simulink model "sim660"  (R2025a)
settings: Solver=ode23s  StartTime=0.0  StopTime=10000  RelTol=1e-3
model workspace (MAT data in the model file):
  op_snapshot1 : opcond.OperatingPoint (value not decoded)
undefined symbols (not defined in the file or in its folder): State132MW, State198MW, State198MW_DELAY
libraries: slpidlib x4, simulink x2, adrc_toolbox_library x1
(part 4 of 5)

== matlab function sim660/Subsystem/MATLAB Function ==
  data: Qc input; Dfw input; dpm output; Dst input; hst input; Drc input; hfw input; pm input; hm input; dhm output; dH output; Vm input; Cm input; eff input; state output; S input; H input; drhodp output; drhodh output; dTdp output; dTdh output; dhVdp output; dhLdp output; drhoVdp output; drhoLdp output; dxdp output; dxdh output
function [dpm,dhm,dH,state,drhodp,drhodh,dTdp,dTdh,dhVdp,dhLdp,drhoVdp,drhoLdp,dxdp,dxdh] = fcn(Qc,Dfw,Dst,hst,Drc,hfw,pm,hm,Vm,Cm,eff,S,H)
%Vm=10;
%Cm=2000;
%eff=0.9;
x=x_ph(pm,hm);
rho=rho_ph(pm,hm);

%%%%%干湿态分别算
if not (x<1 && x>0)
    state=1;
    drhodp=diffx(@rho_ph,pm,hm);
    drhodh=diffy(@rho_ph,pm,hm);
    dTdp=diffx(@T_ph,pm,hm);
    dTdh=diffy(@T_ph,pm,hm);
    A=Vm*drhodp;
    B=Vm*drhodh;
    C=Vm*hm*drhodp+Cm*dTdp;
    D=Vm*hm*drhodh+Vm*rho+Cm*dTdh;
    E=Dfw-Dst;
    F=Dfw*hfw-Dst*hst+Qc;
    out=[A B;C D]\[E;F];
    dpm=out(1);
    dhm=out(2);
    dhVdp=nan;
    dhLdp=nan;
    drhoVdp=nan;
    drhoLdp=nan;
    dxdp=nan;
    dxdh=nan;
    if H>0
        vL=vL_p(pm);
        rhoL=1/vL;
        dH=(-Dst+Dfw+Drc)/(S*rhoL);
    else
    dH=0;
    end
else
    state=x;
    vV=vV_p(pm);
    vL=vL_p(pm);
    rhoV=1/vV;
    rhoL=1/vL;
    hV=hV_p(pm);
    hL=hL_p(pm);
    dTdp=diff1(@Tsat_p,pm);
    dhVdp=dhVdp_p(pm);
    dhLdp=dhLdp_p(pm);
    drhoVdp=diff1(@rho_Vp,pm);
    drhoLdp=diff1(@rho_Lp,pm);
    dxdp=diffx(@x_ph,pm,hm);
    dxdh=diffy(@x_ph,pm,hm);
    %https://www.sciencedirect.com/science/article/pii/S1359431116327727
    Dx=(1-x)*(Dfw+Drc)*eff;
    %A=Vm*(x*drhoVdp+rhoV*dxdp+((1-x)*drhoLdp-rhoL*dxdp)*(1-eff));
    A=Vm*(x*drhoVdp+rhoV*dxdp+((1-x)*drhoLdp-rhoL*dxdp));
    B=Vm*(rhoV*dxdh-rhoL*dxdh);

    %C=Vm*hV*(x*drhoVdp+rhoV*dxdp)+(Vm*hL*((1-x)*drhoLdp-rhoL*dxdp)+Vm*rhoV*x*dhVdp+Vm*rhoL*(1-x)*dhLdp)*(1-eff)+Cm*dTdp;
    C=Vm*hV*(x*drhoVdp+rhoV*dxdp)+(Vm*hL*((1-x)*drhoLdp-rhoL*dxdp)+Vm*rhoV*x*dhVdp+Vm*rhoL*(1-x)*dhLdp)+Cm*dTdp;
    D=Vm*hV*rhoV*dxdh-Vm*hL*rhoL*dxdh;
   
    E=Dfw-Dst+Drc-Dx;
    F=Dfw*hfw+Drc*hL-Dx*hL-Dst*hst+Qc;

    out =[A B;C D]\[E;F];
    dpm=out(1);
    dhm=out(2);
    %dH=(Vm*((1-x)*drhoLdp*dpm-rhoL*dxdh*dhm-rhoL*dxdp*dpm)*eff-Drc)/S;
    dH=(Dx-Drc)/(S*rhoL);
    drhodp=nan;
    drhodh=nan;
    dTdh=nan;

end

%[a b;c d][dpm;dhm]=[e;f]
%out=[dpm;dhm]


end

%%IF97


function rho=rho_Vp(p)
rho=1/vV_p(p);
end
function rho=rho_Lp(p)
rho=1/vL_p(p);
end
function rho=rho_ph(p,h)

rho=1/v_ph(p,h);
end
%% quality
function x = x_ph(p,h)
x = (h - hL_p(p))./(hV_p(p) - hL_p(p));
end

%% stand alone functions
function dhLdp = dhLdp_p(p)
% dhLdp = dhLdp_ph(p)
%   Derivative of enthalpy wrt pressure of saturated liquid, dhLdp [(kJ/kg)/MPa], as a function of pressure, p [MPa]
% based on IAPWS-IF97
% Reference: http://www.iapws.org/
% June 16, 2009
% Mark Mikofski
%% size of inputs
dim = size(p);
dhLdp = NaN(dim);
%% constants and calculated
conversion_factor = 1e-3; % [MPa/(kJ/m^3)]
Tmin = 273.16; % [K] minimum temperature is triple point
TB13 = 623.15; % [K] temperature at boundary between region 1 and 3
pmin = psat_T(Tmin); % [MPa] minimum pressure is 611.657 Pa
pB13sat = psat_T(TB13); % [MPa] saturation pressure at boundary between region 1 and 3, 16.5291643 MPa
pc = 22.064; % [MPa] critical pressure
Tsat = Tsat_p(p); % [K] saturation temperatures
%% valid ranges
valid4a = p>=pmin & p<=pB13sat; % valid range for saturated liquid in region 4a
valid4b = p>pB13sat & p<=pc; % valid range for saturated liquid in region 4b
if any(any(valid4a))
    p4a = p(valid4a);Tsat4a = Tsat(valid4a);
    dhLdp(valid4a) = v1_pT(p4a,Tsat4a).*(1-Tsat4a.*alphav1_pT(p4a,Tsat4a))/conversion_factor + cp1_pT(p4a,Tsat4a).*dTsatdpsat_p(p4a); % [(kJ/kg)/MPa]
end
if any(any(valid4b))
    p4b = p(valid4b); Tsat4b = Tsat(valid4b);v3L = vL_p(p4b);rho3L = 1./v3L;dTsatdpsat4b = dTsatdpsat_p(p4b);
    betap3L = betap3_rhoT(rho3L,Tsat4b);alphap3L = alphap3_rhoT(rho3L,Tsat4b);cv3L = cv3_rhoT(rho3L,Tsat4b);
    dhLdp(valid4b) = (v3L - Tsat4b.*alphap3L./betap3L.*(1 - p4b.*alphap3L.*dTsatdpsat4b))/conversion_factor + (cv3L + p4b.*v3L.*alphap3L).*dTsatdpsat4b;
end
end
function dhVdp = dhVdp_p(p)
% dhVdp = dhVdp_ph(p)
%   Derivative of enthalpy wrt pressure of saturated vapor, dhVdp [(kJ/kg)/MPa], as a function of pressure, p [MPa]
% based on IAPWS-IF97
% Reference: http://www.iapws.org/
% June 16, 2009
% Mark Mikofski
%% size of inputs
dim = size(p);
dhVdp = NaN(dim);
%% constants and calculated
conversion_factor = 1e-3; % [MPa/(kJ/m^3)]
Tmin = 273.16; % [K] minimum temperature is triple point
TB13 = 623.15; % [K] temperature at boundary between region 1 and 3
pmin = psat_T(Tmin); % [MPa] minimum pressure is 611.657 Pa
pB13sat = psat_T(TB13); % [MPa] saturation pressure at boundary between region 1 and 3, 16.5291643 MPa
pc = 22.064; % [MPa] critical pressure
Tsat = Tsat_p(p); % [K] saturation temperatures
%% valid ranges
valid4a = p>=pmin & p<=pB13sat; % valid range for saturated liquid in region 4a
valid4b = p>pB13sat & p<=pc; % valid range for saturated liquid in region 4b
if any(any(valid4a))
    p4a = p(valid4a);Tsat4a = Tsat(valid4a);
    dhVdp(valid4a) = v2_pT(p4a,Tsat4a).*(1-Tsat4a.*alphav2_pT(p4a,Tsat4a))/conversion_factor + cp2_pT(p4a,Tsat4a).*dTsatdpsat_p(p4a); % [(kJ/kg)/MPa]
end
if any(any(valid4b))
    p4b = p(valid4b); Tsat4b = Tsat(valid4b);v3V = vV_p(p4b);rho3V = 1./v3V;dTsatdpsat4b = dTsatdpsat_p(p4b);
    betap3V = betap3_rhoT(rho3V,Tsat4b);alphap3V = alphap3_rhoT(rho3V,Tsat4b);cv3V = cv3_rhoT(rho3V,Tsat4b);
    dhVdp(valid4b) = (v3V - Tsat4b.*alphap3V./betap3V.*(1 - p4b.*alphap3V.*dTsatdpsat4b))/conversion_factor + (cv3V + p4b.*v3V.*alphap3V).*dTsatdpsat4b;
end
end
function v = vL_p(p)
% v = vL_p(p)
%   Specific volume of saturated liquid, v [m^3/kg], as a function of pressure, p [MPa]
% based on IAPWS-IF97
% Reference: http://www.iapws.org/
% June 5, 2009
% Mark Mikofski
%% size of inputs
dim = size(p);
v = NaN(dim);
%% constants and calculated
Tmin = 273.16; % [K] minimum temperature is triple point
TB13 = 623.15; % [K] temperature at boundary between region 1 and 3
pmin = psat_T(Tmin); % [MPa] minimum pressure is 611.657 Pa
pB13sat = psat_T(TB13); % [MPa] saturation pressure at boundary between region 1 and 3, 16.5291643 MPa
pc = 22.064; % [MPa] critical pressure
Tsat = Tsat_p(p); % [K] saturation temperatures
%% valid ranges
valid4a = p>=pmin & p<=pB13sat; % valid range for saturated liquid in region 4a
valid4b = p>pB13sat & p<=pc; % valid range for saturated liquid in region 4b
if any(any(valid4a))
    v(valid4a) = v1_pT(p(valid4a),Tsat(valid4a)); % [kJ/kg] saturated liquid enthalpies in region 1
end
if any(any(valid4b))
    p3cd = 19.00881189173929; % [MPa] pressure given by T3cd_p(p) = Tsat_p(p)
    valid3c = p>pB13sat & p<=p3cd;
    p3q = psat_T(643.15); % [MPa] 21.0434 MPa
    valid3s = p>p3cd & p<=p3q;
    p3y = 21.93161551; % [MPa] p3sat_v(0.00264 m^3/kg), n.b. p3sat_v is not an available function yet
    valid3u = p>p3q & p<=p3y;
    valid3y = p>p3y & p<=pc;
    if any(any(valid3c))
        v(valid3c) = v3c_pT(p(valid3c),Tsat(valid3c));
    end
    if any(any(valid3s))
        v(valid3s) = v3s_pT(p(valid3s),Tsat(valid3s));
    end
    if any(any(valid3u))
        v(valid3u) = v3u_pT(p(valid3u),Tsat(valid3u));
    end
    if any(any(valid3y))
        v(valid3y) = v3y_pT(p(valid3y),Tsat(valid3y));
    end
end
end
function v = vV_p(p)
% v = vV_p(p)
%   Specific volume of saturated vapor, v [m^3/kg], as a function of pressure, p [MPa]
% based on IAPWS-IF97
% Reference: http://www.iapws.org/
% June 5, 2009
% Mark Mikofski
%% size of inputs
dim = size(p);
v = NaN(dim);
%% constants and calculated
Tmin = 273.16; % [K] minimum temperature is triple point
TB13 = 623.15; % [K] temperature at boundary between region 1 and 3
pmin = psat_T(Tmin); % [MPa] minimum pressure is 611.657 Pa
pB13sat = psat_T(TB13); % [MPa] saturation pressure at boundary between region 1 and 3, 16.5291643 MPa
pc = 22.064; % [MPa] critical pressure
Tsat = Tsat_p(p); % [K] saturation temperatures
%% valid ranges
valid4a = p>=pmin & p<=pB13sat; % valid range for saturated liquid in region 4a
valid4b = p>pB13sat & p<=pc; % valid range for saturated liquid in region 4b
if any(any(valid4a))
    v(valid4a) = v2_pT(p(valid4a),Tsat(valid4a)); % [kJ/kg] saturated liquid enthalpies in region 2
end
if any(any(valid4b))
    valid3t = p>pB13sat & p<=20.5;
    p3q = psat_T(643.15); % [MPa] 21.0434 MPa
    valid3r = p>20.5 & p<=p3q;
    p3z = 21.90096265; % [MPa] p3sat_v(0.00385 m^3/kg), n.b. p3sat_v is not an available function yet
    valid3x = p>p3q & p<=p3z;
    valid3z = p>p3z & p<=pc;
    if any(any(valid3t))
        v(valid3t) = v3t_pT(p(valid3t),Tsat(valid3t));
    end
    if any(any(valid3r))
        v(valid3r) = v3r_pT(p(valid3r),Tsat(valid3r));
    end
    if any(any(valid3x))
        v(valid3x) = v3x_pT(p(valid3x),Tsat(valid3x));
    end
    if any(any(valid3z))
        v(valid3z) = v3z_pT(p(valid3z),Tsat(valid3z));
    end
end
end
function h = hL_p(p)
% h = hL_p(p)
%   Enthalpy of saturated liquid, h [kJ/kg], as a function of pressure, p [MPa]
% based on IAPWS-IF97
% Reference: http://www.iapws.org/
% June 2, 2009
% Mark Mikofski
%% size of inputs
dim = size(p);
h = NaN(dim);
%% constants and calculated
Tmin = 273.16; % [K] minimum temperature is triple point
TB13 = 623.15; % [K] temperature at boundary between region 1 and 3
pmin = psat_T(Tmin); % [MPa] minimum pressure is 611.657 Pa
pB13sat = psat_T(TB13); % [MPa] saturation pressure at boundary between region 1 and 3, 16.5291643 MPa
pc = 22.064; % [MPa] critical pressure
Tsat = Tsat_p(p); % [K] saturation temperatures
%% valid ranges
valid4a = p>=pmin & p<=pB13sat; % valid range for saturated liquid in region 4a
valid4b = p>pB13sat & p<=pc; % valid range for saturated liquid in region 4b
if any(any(valid4a))
    h(valid4a) = h1_pT(p(valid4a),Tsat(valid4a)); % [kJ/kg] saturated liquid enthalpies in region 1
end
if any(any(valid4b))
    h(valid4b) = h3_rhoT(1./vL_p(p(valid4b)),Tsat(valid4b));
end
end
function h = hV_p(p)
% h = hV_p(p)
%   Enthalpy of saturated vapor, h [kJ/kg], as a function of pressure, p [MPa]
% based on IAPWS-IF97
% Reference: http://www.iapws.org/
% June 2, 2009
% Mark Mikofski
%% size of inputs
dim = size(p);
h = NaN(dim);
%% constants and calculated
Tmin = 273.16; % [K] minimum temperature is triple point
TB13 = 623.15; % [K] temperature at boundary between region 1 and 3
pmin = psat_T(Tmin); % [MPa] minimum pressure is 611.657 Pa
pB13sat = psat_T(TB13); % [MPa] saturation pressure at boundary between region 1 and 3, 16.5291643 MPa
pc = 22.064; % [MPa] critical pressure
Tsat = Tsat_p(p); % [K] saturation temperatures
%% valid ranges
valid4a = p>=pmin & p<=pB13sat; % valid range for saturated liquid in region 4a
valid4b = p>pB13sat & p<=pc; % valid range for saturated liquid in region 4b
if any(any(valid4a))
    h(valid4a) = h2_pT(p(valid4a),Tsat(valid4a)); % [kJ/kg] saturated liquid enthalpies in region 2
end
if any(any(valid4b))
    h(valid4b) = h3_rhoT(1./vV_p(p(valid4b)),Tsat(valid4b));
end
end
function T = T_ph(p,h)
% T = T_ph(p,h)
%   Temperature of liquid, vapor or mixture, T [K], as functions of pressure, p [MPa], and enthalpy, h [kJ/kg]
% based on IAPWS-IF97
% Reference: http://www.iapws.org/
% June 2, 2009
% Mark Mikofski
%% size of inputs
dim = size(p);
initnan = NaN(dim);
T = initnan;
%% constants and calculated scalars
Tmin = 273.16; % [K] minimum temperature is triple point
T2bcsat = 554.485; % [K] saturation temperature at 5.85 kJ/kg/K isentropic line between region 2b and 2c
TB13 = 623.15; % [K] temperature at boundary between region 1 and 3
Tmax = 1073.15; % [K] maximum temperature
pmin = psat_T(Tmin); % [MPa] minimum pressure is 611.657 Pa
p2ab = 4; % [MPa] pressure along boundary between region 2a and 2b
p2bcsat = psat_T(T2bcsat); % [MPa] saturation pressure at 5.85 kJ/kg/K isentropic line between region 2b and 2c
pB13sat = psat_T(TB13); % [MPa] saturation pressure at boundary between region 1 and 3, 16.5291643 MPa
pmax = 100; % [MPa] maximum pressure
h1B13L = h1_pT(pB13sat,TB13); % [kJ/kg] saturated liquid enthalpy at boundary between region 1, region 3 and region 4
h2B13V = h2_pT(pB13sat,TB13); % [kJ/kg] saturated vapor enthalpy at boundary between region 2, region 3 and region 4
%% calculated matrices
Tsat = Tsat_p(p); % [K] saturation temperatures
h1min = initnan;h2max = initnan;valid = p>=pmin & p<=pmax;pvalid = p(valid); % initialize matricies with NaN and set valid range of parameters
if any(any(valid))
    Tmin = Tmin*ones(dim);Tmax = Tmax*ones(dim); % copy to matrix of size dim
    h1min(valid) = h1_pT(pvalid,Tmin(valid)); % [kJ/kg] minimum enthalpies
    h2max(valid) = h2_pT(pvalid,Tmax(valid)); % [kJ/kg] maximum enthalpies in region 2
end
h1L = initnan;h2V = initnan;valid = p>=pmin & p<=pB13sat;pvalid = p(valid); % initialize matricies with NaN and set valid range of parameters
if any(any(valid))
    h1L(valid) = h1_pT(pvalid,Tsat(valid)); % [kJ/kg] saturated liquid enthalpies in region 1
    h2V(valid) = h2_pT(pvalid,Tsat(valid)); % [kJ/kg] saturated vapor enthalpies in region 2
end
h1B13 = initnan;h3ab = initnan;h2B23 = initnan;valid = p>=pB13sat & p<=pmax;pvalid = p(valid); % initialize matricies with NaN and set valid range of parameters
if any(any(valid))
    TB13 = TB13*ones(dim); % copy to matrix of size dim
    h1B13(valid) = h1_pT(pvalid,TB13(valid)); % [kJ/kg] enthalpies on boundary between region 1 and region 3
    h3ab(valid) = h3ab_p(pvalid); % [kJ/kg] enthalpies on critical entropy isentropic line between regions 3a and region 3b
    h2B23(valid) = h2_pT(pvalid,TB23_p(pvalid)); % [kJ/kg] enthalpies on boundary between region 2 and region 3
end
h2bc = initnan;valid = p>=p2bcsat & p<=pmax; % initialize matricies with NaN and set valid range of parameters
h2bc(valid) = h2bc_p(p(valid)); % [kJ/kg] enthalpies on boundary between region 2b and 2c
p3sat = pB13sat*ones(dim);valid = h>=h1B13L & h<=h2B13V; % % do NOT use NaN to initialize p3sat, b/c for h<h1B13L or h>h2B13V p>NaN = 0, instead use pB13sat
if any(any(valid))
    p3sat(valid) = p3sat_h(h(valid)); % [MPa] saturation pressure on boundary between region 3 and 4
end
%% valid ranges
valid1 = (p>=pmin & p<=pB13sat & h>=h1min & h<=h1L) | (p>pB13sat & p<=pmax & h>=h1min & h<=h1B13); % valid range for region 1
valid2a = p>=pmin & p<=p2ab & h>h2V & h<=h2max; % valid range for region 2a
valid2b = (p>p2ab & p<=p2bcsat & h>h2V & h<=h2max) | (p>p2bcsat & p<=pmax & h>h2bc & h<=h2max); % valid range for region 2b
valid2c = (p>p2bcsat & p<=pB13sat & h>h2V & h<=h2bc) | (p>pB13sat & p<=pmax & h>h2B23 & h<=h2bc); % valid range for region 2c
valid3a = p>p3sat & p<=pmax & h>h1B13 & h<=h3ab; % valid range for region 3a
valid3b = p>p3sat & p<=pmax & h>h3ab & h<=h2B23; % valid range for region 3b
valid4 = (p>=pmin & p<=pB13sat & h>h1L & h<=h2V) | (p>pB13sat & p<=p3sat & h>h1B13L & h<=h2B13V); % valid range for region 4
if any(any(valid1))
    T(valid1) = T1_ph(p(valid1),h(valid1));
end
if any(any(valid2a))
    T(valid2a) = T2a_ph(p(valid2a),h(valid2a));
end
if any(any(valid2b))
    T(valid2b) = T2b_ph(p(valid2b),h(valid2b));
end
if any(any(valid2c))
    T(valid2c) = T2c_ph(p(valid2c),h(valid2c));
end
if any(any(valid3a))
    T(valid3a) = T3a_ph(p(valid3a),h(valid3a));
end
if any(any(valid3b))
    T(valid3b) = T3b_ph(p(valid3b),h(valid3b));
end
if any(any(valid4))
    T(valid4) = Tsat(valid4);
end
end
function v = v_ph(p,h)
% v = v_ph(p,h)
%   Specific volume of liquid, vapor or mixture, v [m^3/kg], as functions of pressure, p [MPa], and enthalpy, h [kJ/kg]
% based on IAPWS-IF97
% Reference: http://www.iapws.org/
% June 1, 2009
% Mark Mikofski
%% size of inputs
dim = size(p);
initnan = NaN(dim);
v = initnan;
%% constants and calculated scalars
Tmin = 273.16; % [K] minimum temperature is triple point
T2bcsat = 554.485; % [K] saturation temperature at 5.85 kJ/kg/K isentropic line between region 2b and 2c
TB13 = 623.15; % [K] temperature at boundary between region 1 and 3
Tmax = 1073.15; % [K] maximum temperature
pmin = psat_T(Tmin); % [MPa] minimum pressure is 611.657 Pa
p2ab = 4; % [MPa] pressure along boundary between region 2a and 2b
p2bcsat = psat_T(T2bcsat); % [MPa] saturation pressure at 5.85 kJ/kg/K isentropic line between region 2b and 2c
pB13sat = psat_T(TB13); % [MPa] saturation pressure at boundary between region 1 and 3, 16.5291643 MPa
pmax = 100; % [MPa] maximum pressure
h1B13L = h1_pT(pB13sat,TB13); % [kJ/kg] saturated liquid enthalpy at boundary between region 1, region 3 and region 4
h2B13V = h2_pT(pB13sat,TB13); % [kJ/kg] saturated vapor enthalpy at boundary between region 2, region 3 and region 4
%% calculated matrices
Tsat = Tsat_p(p); % [K] saturation temperatures
h1min = initnan;h2max = initnan;valid = p>=pmin & p<=pmax;pvalid = p(valid); % initialize matricies with NaN and set valid range of parameters
if any(any(valid))
    Tmin = Tmin*ones(dim);Tmax = Tmax*ones(dim); % copy to matrix of size dim
    h1min(valid) = h1_pT(pvalid,Tmin(valid)); % [kJ/kg] minimum enthalpies
    h2max(valid) = h2_pT(pvalid,Tmax(valid)); % [kJ/kg] maximum enthalpies in region 2
end
h1L = initnan;h2V = initnan;valid = p>=pmin & p<=pB13sat;pvalid = p(valid); % initialize matricies with NaN and set valid range of parameters
if any(any(valid))
    h1L(valid) = h1_pT(pvalid,Tsat(valid)); % [kJ/kg] saturated liquid enthalpies in region 1
    h2V(valid) = h2_pT(pvalid,Tsat(valid)); % [kJ/kg] saturated vapor enthalpies in region 2
end
h1B13 = initnan;h3ab = initnan;h2B23 = initnan;valid = p>=pB13sat & p<=pmax;pvalid = p(valid); % initialize matricies with NaN and set valid range of parameters
if any(any(valid))
    TB13 = TB13*ones(dim); % copy to matrix of size dim
    h1B13(valid) = h1_pT(pvalid,TB13(valid)); % [kJ/kg] enthalpies on boundary between region 1 and region 3
    h3ab(valid) = h3ab_p(pvalid); % [kJ/kg] enthalpies on critical entropy isentropic line between regions 3a and region 3b
    h2B23(valid) = h2_pT(pvalid,TB23_p(pvalid)); % [kJ/kg] enthalpies on boundary between region 2 and region 3
end
h2bc = initnan;valid = p>=p2bcsat & p<=pmax; % initialize matricies with NaN and set valid range of parameters
h2bc(valid) = h2bc_p(p(valid)); % [kJ/kg] enthalpies on boundary between region 2b and 2c
p3sat = pB13sat*ones(dim);valid = h>=h1B13L & h<=h2B13V; % % do NOT use NaN to initialize p3sat, b/c for h<h1B13L or h>h2B13V p>NaN = 0, instead use pB13sat
if any(any(valid))
    p3sat(valid) = p3sat_h(h(valid)); % [MPa] saturation pressure on boundary between region 3 and 4
end
%% valid ranges
valid1 = (p>=pmin & p<=pB13sat & h>=h1min & h<=h1L) | (p>pB13sat & p<=pmax & h>=h1min & h<=h1B13); % valid range for region 1
valid2a = p>=pmin & p<=p2ab & h>h2V & h<=h2max; % valid range for region 2a
valid2b = (p>p2ab & p<=p2bcsat & h>h2V & h<=h2max) | (p>p2bcsat & p<=pmax & h>h2bc & h<=h2max); % valid range for region 2b
valid2c = (p>p2bcsat & p<=pB13sat & h>h2V & h<=h2bc) | (p>pB13sat & p<=pmax & h>h2B23 & h<=h2bc); % valid range for region 2c
valid3a = p>p3sat & p<=pmax & h>h1B13 & h<=h3ab; % valid range for region 3a
valid3b = p>p3sat & p<=pmax & h>h3ab & h<=h2B23; % valid range for region 3b
valid4a = p>=pmin & p<=pB13sat & h>h1L & h<=h2V; % valid range for region 4a
valid4b = p>pB13sat & p<=p3sat & h>h1B13L & h<=h2B13V; % valid range for region 4b
if any(any(valid1))
    p1 = p(valid1);
    v(valid1) = v1_pT(p1,T1_ph(p1,h(valid1)));
end
if any(any(valid2a))
    p2a = p(valid2a);
    v(valid2a) = v2_pT(p2a,T2a_ph(p2a,h(valid2a)));
end
if any(any(valid2b))
    p2b = p(valid2b);
    v(valid2b) = v2_pT(p2b,T2b_ph(p2b,h(valid2b)));
end
if any(any(valid2c))
    p2c = p(valid2c);
    v(valid2c) = v2_pT(p2c,T2c_ph(p2c,h(valid2c)));
end
if any(any(valid3a))
    v(valid3a) = v3a_ph(p(valid3a),h(valid3a));
end
if any(any(valid3b))
    v(valid3b) = v3b_ph(p(valid3b),h(valid3b));
end
if any(any(valid4a))
    p4a = p(valid4a);Tsat4a = Tsat(valid4a);h1L4a = h1L(valid4a);
    x = (h(valid4a)-h1L4a)./(h2V(valid4a)-h1L4a); % quality
    v1L = v1_pT(p4a,Tsat4a); % [m^3/kg] saturated liquid specific volumes
    v2V = v2_pT(p4a,Tsat4a); % [m^3/kg] saturated vapor specific volumes
    v(valid4a) = v1L + x.*(v2V - v1L);
end
if any(any(valid4b))
    p4b = p(valid4b); Tsat4b = Tsat(valid4b);
    v3L = vL_p(p4b); v3V = vV_p(p4b);
    h3L = h3_rhoT(1./v3L,Tsat4b);
    h3V = h3_rhoT(1./v3V,Tsat4b);
    x = (h(valid4b)-h3L)./(h3V-h3L); % quality
    v(valid4b) = v3L + x.*(v3V - v3L);
end
end
function p = psat_T(T)
% p = psat_T(T)
%   Pressure of saturated liquid, mixture or steam, p [MPa], as a function of temperature, T [K]
% based on IAPWS-IF97
% Reference: http://www.iapws.org/
% June 9, 2009
% Mark Mikofski
dim = size(T);
p = NaN(dim);
Tmin = 273.16; % [K] minimum temperature is triple point
Tc = 647.096; % [K] critical point temperature
valid = T>=Tmin & T<=Tc;
pstar = 1; % [Mpa]
Tstar = 1; % [K]
n = [1167.05214527670;-724213.167032060;-17.0738469400920;12020.8247024700;-3232555.03223330;14.9151086135300; ...
    -4823.26573615910;405113.405420570;-0.238555575678490;650.175348447980];
upsilon = T(valid)/Tstar + n(9)./(T(valid)/Tstar-n(10));
A = (upsilon + n(1)).*upsilon + n(2); % use Horner's Method to speed up calculations
B = (n(3)*upsilon + n(4)).*upsilon + n(5); % use Horner's Method to speed up calculations
C = (n(6)*upsilon + n(7)).*upsilon + n(8); % use Horner's Method to speed up calculations
beta = 2*C./(-B + (B.^2 - 4*A.*C).^0.5);
p(valid) = (beta.^4) * pstar;
end
function T = Tsat_p(p)
% T = Tsat_p(p)
%   Temperature of saturated liquid, mixture or steam, T [K], as a function of temperature, p [MPa]
% based on IAPWS-IF97
% Reference: http://www.iapws.org/
% June 9, 2009
% Mark Mikofski
dim = size(p);
T = NaN(dim);
Tmin = 273.16; % [K] minimum temperature is triple point
pmin = psat_T(Tmin); % [MPa] minimum pressure is 611.657 Pa
pc = 22.064; % [MPa] critical pressure
valid = p>=pmin & p<=pc; % initialize matricies with NaN and set valid range of parameters
pstar = 1; % [Mpa]
Tstar = 1; % [K]
n = [1167.05214527670;-724213.167032060;-17.0738469400920;12020.8247024700;-3232555.03223330;14.9151086135300; ...
    -4823.26573615910;405113.405420570;-0.238555575678490;650.175348447980];
beta = (p(valid)/pstar).^0.25;
E = (beta + n(3)).*beta + n(6); % use Horner's Method to speed up calculations
F = (n(1)*beta + n(4)).*beta + n(7); % use Horner's Method to speed up calculations
G = (n(2)*beta + n(5)).*beta + n(8); % use Horner's Method to speed up calculations
D = 2*G./(-F - (F.^2 - 4*E.*G).^0.5);
n11 = n(10) + D;
theta = (n11 - (n11.^2 - 4*(n(9) + n(10)*D)).^0.5)/2;
T(valid) = theta*Tstar;
end
%% basic and fundamental functions
function h = h1_pT(p,T) % [kJ/kg]
R = 0.461526; % [kJ/kg/K] specific gas constant
Tstar = 1386; % [K]
h = R*Tstar*dgammadtau1_pT(p,T);
end
function h = h2_pT(p,T) % [kJ/kg]
R = 0.461526; % [kJ/kg/K] specific gas constant
Tstar = 540; % [K]
h = R*Tstar*dgammadtau2_pT(p,T);
end
function h = h3_rhoT(rho,T)
R = 0.461526; % [kJ/kg/K] specific gas constant
Tc = 647.096; % [K] critical point temperature
rhoc = 322; % [kg/m^3] critical point density
delta = rho/rhoc;
h = R*(Tc*dphidtau3_rhoT(rho,T) + T.*delta.*dphiddelta3_rhoT(rho,T));
end
function v = v1_pT(p,T) % [m^3/kg]
R = 0.461526; % [kJ/kg/K] specific gas constant
conversion_factor = 1e-3; % [MPa/(kJ/m^3)]
pstar = 16.53; % [MPa]
v = conversion_factor*R*T/pstar.*dgammadpi1_pT(p,T);
end
function v = v2_pT(p,T) % [m^3/kg]
R = 0.461526; % [kJ/kg/K] specific gas constant
conversion_factor = 1e-3; % [MPa/(kJ/m^3)]
pstar = 1; % [MPa]
v = conversion_factor*R*T/pstar.*dgammadpi2_pT(p,T);
end
function cp = cp1_pT(p,T) % [kJ/kg/K]
R = 0.461526; % [kJ/kg/K] specific gas constant
Tstar = 1386; % [K]
tau = Tstar./T;
cp = -R*tau.^2.*dgammadtautau1_pT(p,T);
end
function cp = cp2_pT(p,T) % [kJ/kg/K]
R = 0.461526; % [kJ/kg/K] specific gas constant
Tstar = 540; % [K]
tau = Tstar./T;
cp = -R*tau.^2.*dgammadtautau2_pT(p,T);
end
function cv = cv3_rhoT(rho,T)
R = 0.461526; % [kJ/kg/K] specific gas constant
Tc = 647.096; % [K] critical point temperature
tau = Tc./T;
cv = R*(-tau.^2.*dphidtautau3_rhoT(rho,T));
end
function alphav = alphav1_pT(p,T)
Tstar = 1386; % [K]
tau = Tstar./T;
alphav = (1-tau.*dgammadpitau1_pT(p,T)./dgammadpi1_pT(p,T))./T;
end
function alphav = alphav2_pT(p,T)
Tstar = 540; % [K]
tau = Tstar./T;
alphav = (1-tau.*dgammadpitau2_pT(p,T)./dgammadpi2_pT(p,T))./T;
end
function alphap = alphap3_rhoT(rho,T)
Tc = 647.096; % [K] critical point temperature
tau = Tc./T;
alphap = (1-tau.*dphiddeltatau3_rhoT(rho,T)./dphiddelta3_rhoT(rho,T))./T;
end
function betap = betap3_rhoT(rho,T)
rhoc = 322; % [kg/m^3] critical point density
delta = rho/rhoc;
betap = rho.*(2+delta.*dphiddeltadelta3_rhoT(rho,T)./dphiddelta3_rhoT(rho,T));
end
function dgammadtau = dgammadtau1_pT(p,T)
dim = length(p);
pstar = 16.53; % [MPa]
Tstar = 1386; % [K]
pi = p/pstar;
tau = Tstar./T;
I = [0,0,0,0,0,0,0,0,1,1,1,1,1,1,2,2,2,2,2,3,3,3,4,4,4,5,8,8,21,23,29,30,31,32];
J = [-2,-1,0,1,2,3,4,5,-9,-7,-1,0,1,3,-3,0,1,3,17,-4,0,6,-5,-2,10,-8,-11,-6,-29,-31,-38,-39,-40,-41];
n = [0.146329712131670,-0.845481871691140,-3.75636036720400,3.38551691683850,-0.957919633878720,0.157720385132280, ...
    -0.0166164171995010,0.000812146299835680,0.000283190801238040,-0.000607063015658740,-0.0189900682184190, ...
    -0.0325297487705050,-0.0218417171754140,-5.28383579699300e-05,-0.000471843210732670,-0.000300017807930260, ...
    4.76613939069870e-05,-4.41418453308460e-06,-7.26949962975940e-16,-3.16796448450540e-05,-2.82707979853120e-06, ...
    -8.52051281201030e-10,-2.24252819080000e-06,-6.51712228956010e-07,-1.43417299379240e-13,-4.05169968601170e-07, ...
    -1.27343017416410e-09,-1.74248712306340e-10,-6.87621312955310e-19,1.44783078285210e-20,2.63357816627950e-23, ...
    -1.19476226400710e-23,1.82280945814040e-24,-9.35370872924580e-26];
Nterms = 34;
I = ones(dim,1)*I;
J = ones(dim,1)*J;
n = ones(dim,1)*n;
pi = pi*ones(1,Nterms);
tau = tau*ones(1,Nterms);
dgammadtau = sum(n.*(7.1-pi).^I.*J.*(tau-1.222).^(J-1),2);
end
function dgammadpi = dgammadpi1_pT(p,T)
dim = length(p);
pstar = 16.53; % [MPa]
Tstar = 1386; % [K]
pi = p/pstar;
tau = Tstar./T;
I = [0,0,0,0,0,0,0,0,1,1,1,1,1,1,2,2,2,2,2,3,3,3,4,4,4,5,8,8,21,23,29,30,31,32];
J = [-2,-1,0,1,2,3,4,5,-9,-7,-1,0,1,3,-3,0,1,3,17,-4,0,6,-5,-2,10,-8,-11,-6,-29,-31,-38,-39,-40,-41];
n = [0.146329712131670,-0.845481871691140,-3.75636036720400,3.38551691683850,-0.957919633878720,0.157720385132280, ...
    -0.0166164171995010,0.000812146299835680,0.000283190801238040,-0.000607063015658740,-0.0189900682184190, ...
    -0.0325297487705050,-0.0218417171754140,-5.28383579699300e-05,-0.000471843210732670,-0.000300017807930260, ...
    4.76613939069870e-05,-4.41418453308460e-06,-7.26949962975940e-16,-3.16796448450540e-05,-2.82707979853120e-06, ...
    -8.52051281201030e-10,-2.24252819080000e-06,-6.51712228956010e-07,-1.43417299379240e-13,-4.05169968601170e-07, ...
    -1.27343017416410e-09,-1.74248712306340e-10,-6.87621312955310e-19,1.44783078285210e-20,2.63357816627950e-23, ...
    -1.19476226400710e-23,1.82280945814040e-24,-9.35370872924580e-26];
Nterms = 34;
I = ones(dim,1)*I;
J = ones(dim,1)*J;
n = ones(dim,1)*n;
pi = pi*ones(1,Nterms);
tau = tau*ones(1,Nterms);
dgammadpi = sum(-n.*I.*(7.1-pi).^(I-1).*(tau-1.222).^J,2);
end
function dgammadtautau = dgammadtautau1_pT(p,T)
dim = length(p);
pstar = 16.53; % [MPa]
Tstar = 1386; % [K]
pi = p/pstar;
tau = Tstar./T;
I = [0,0,0,0,0,0,0,0,1,1,1,1,1,1,2,2,2,2,2,3,3,3,4,4,4,5,8,8,21,23,29,30,31,32];
J = [-2,-1,0,1,2,3,4,5,-9,-7,-1,0,1,3,-3,0,1,3,17,-4,0,6,-5,-2,10,-8,-11,-6,-29,-31,-38,-39,-40,-41];
n = [0.146329712131670,-0.845481871691140,-3.75636036720400,3.38551691683850,-0.957919633878720,0.157720385132280, ...
    -0.0166164171995010,0.000812146299835680,0.000283190801238040,-0.000607063015658740,-0.0189900682184190, ...
    -0.0325297487705050,-0.0218417171754140,-5.28383579699300e-05,-0.000471843210732670,-0.000300017807930260, ...
    4.76613939069870e-05,-4.41418453308460e-06,-7.26949962975940e-16,-3.16796448450540e-05,-2.82707979853120e-06, ...
    -8.52051281201030e-10,-2.24252819080000e-06,-6.51712228956010e-07,-1.43417299379240e-13,-4.05169968601170e-07, ...
    -1.27343017416410e-09,-1.74248712306340e-10,-6.87621312955310e-19,1.44783078285210e-20,2.63357816627950e-23, ...
    -1.19476226400710e-23,1.82280945814040e-24,-9.35370872924580e-26];
Nterms = 34;
I = ones(dim,1)*I;
J = ones(dim,1)*J;
n = ones(dim,1)*n;
pi = pi*ones(1,Nterms);
tau = tau*ones(1,Nterms);
dgammadtautau = sum(n.*(7.1-pi).^I.*J.*(J-1).*(tau-1.222).^(J-2),2);
end
function dgammadpitau = dgammadpitau1_pT(p,T)
dim = length(p);
pstar = 16.53; % [MPa]
Tstar = 1386; % [K]
pi = p/pstar;
tau = Tstar./T;
I = [0,0,0,0,0,0,0,0,1,1,1,1,1,1,2,2,2,2,2,3,3,3,4,4,4,5,8,8,21,23,29,30,31,32];
J = [-2,-1,0,1,2,3,4,5,-9,-7,-1,0,1,3,-3,0,1,3,17,-4,0,6,-5,-2,10,-8,-11,-6,-29,-31,-38,-39,-40,-41];
n = [0.146329712131670,-0.845481871691140,-3.75636036720400,3.38551691683850,-0.957919633878720,0.157720385132280, ...
    -0.0166164171995010,0.000812146299835680,0.000283190801238040,-0.000607063015658740,-0.0189900682184190, ...
    -0.0325297487705050,-0.0218417171754140,-5.28383579699300e-05,-0.000471843210732670,-0.000300017807930260, ...
    4.76613939069870e-05,-4.41418453308460e-06,-7.26949962975940e-16,-3.16796448450540e-05,-2.82707979853120e-06, ...
    -8.52051281201030e-10,-2.24252819080000e-06,-6.51712228956010e-07,-1.43417299379240e-13,-4.05169968601170e-07, ...
    -1.27343017416410e-09,-1.74248712306340e-10,-6.87621312955310e-19,1.44783078285210e-20,2.63357816627950e-23, ...
    -1.19476226400710e-23,1.82280945814040e-24,-9.35370872924580e-26];
Nterms = 34;
I = ones(dim,1)*I;
J = ones(dim,1)*J;
n = ones(dim,1)*n;
pi = pi*ones(1,Nterms);
tau = tau*ones(1,Nterms);
dgammadpitau = sum(-n.*I.*(7.1-pi).^(I-1).*J.*(tau-1.222).^(J-1),2);
end
function dgammadtau = dgammadtau2_pT(p,T)
dim = length(p);
pstar = 1; % [MPa] scaling pressure for nondimensional pressure, pi
Tstar = 540; % [K] scaling temperature for nondimensional temperature substitution variable
pi = p/pstar; % nondimensional pressure
tau = Tstar./T; % temperature substitution variable
%% ideal part
J0 = [0,1,-5,-4,-3,-2,-1,2,3]; % ideal part exponenets
n0 = [-9.69276865002170,10.0866559680180,-0.00560879112830200,0.0714527380814550,-0.407104982239280,1.42408191714440, ...
    -4.38395113194500,-0.284086324607720,0.0212684637533070];
N0terms = 9; % number of ideal terms in summation
J0 = ones(dim,1)*J0;
n0 = ones(dim,1)*n0;
tau0 = tau*ones(1,N0terms);
dgammadtau0 = sum(n0.*J0.*tau0.^(J0-1),2); % index sums of valid inputs into corresponding location in output array
%% residual part
IR = [1,1,1,1,1,2,2,2,2,2,3,3,3,3,3,4,4,4,5,6,6,6,7,7,7,8,8,9,10,10,10,16,16,18,20,20,20,21,22,23,24,24,24];
JR = [0,1,2,3,6,1,2,4,7,36,0,1,3,6,35,1,2,3,7,3,16,35,0,11,25,8,36,13,4,10,14,29,50,57,20,35,48,21,53,39,26,40,58];
nR = [-0.00177317424732130,-0.0178348622923580,-0.0459960136963650,-0.0575812590834320,-0.0503252787279300, ...
    -3.30326416702030e-05,-0.000189489875163150,-0.00393927772433550,-0.0437972956505730,-2.66745479140870e-05, ...
    2.04817376923090e-08,4.38706672844350e-07,-3.22776772385700e-05,-0.00150339245421480,-0.0406682535626490, ...
    -7.88473095593670e-10,1.27907178522850e-08,4.82253727185070e-07,2.29220763376610e-06,-1.67147664510610e-11, ...
    -0.00211714723213550,-23.8957419341040,-5.90595643242700e-18,-1.26218088991010e-06,-0.0389468424357390, ...
    1.12562113604590e-11,-8.23113408979980,1.98097128020880e-08,1.04069652101740e-19,-1.02347470959290e-13, ...
    -1.00181793795110e-09,-8.08829086469850e-11,0.106930318794090,-0.336622505741710,8.91858453554210e-25, ...
    3.06293168762320e-13,-4.20024676982080e-06,-5.90560296856390e-26,3.78269476134570e-06,-1.27686089346810e-15, ...
    7.30876105950610e-29,5.54147153507780e-17,-9.43697072412100e-07];
NRterms = 43;
IR = ones(dim,1)*IR;
JR = ones(dim,1)*JR;
nR = ones(dim,1)*nR;
pi = pi*ones(1,NRterms);
tauR = tau*ones(1,NRterms);
dgammadtauR = sum(nR.*pi.^IR.*JR.*(tauR-0.5).^(JR-1),2);
dgammadtau = dgammadtau0 + dgammadtauR;
end
function dgammadpi = dgammadpi2_pT(p,T)
dim = length(p);
pstar = 1; % [MPa] scaling pressure for nondimensional pressure, pi
Tstar = 540; % [K] scaling temperature for nondimensional temperature substitution variable
pi = p/pstar; % nondimensional pressure
tau = Tstar./T; % temperature substitution variable
%% ideal part
dgammadpi0 = 1./pi;
%% residual part
IR = [1,1,1,1,1,2,2,2,2,2,3,3,3,3,3,4,4,4,5,6,6,6,7,7,7,8,8,9,10,10,10,16,16,18,20,20,20,21,22,23,24,24,24];
JR = [0,1,2,3,6,1,2,4,7,36,0,1,3,6,35,1,2,3,7,3,16,35,0,11,25,8,36,13,4,10,14,29,50,57,20,35,48,21,53,39,26,40,58];
nR = [-0.00177317424732130,-0.0178348622923580,-0.0459960136963650,-0.0575812590834320,-0.0503252787279300, ...
    -3.30326416702030e-05,-0.000189489875163150,-0.00393927772433550,-0.0437972956505730,-2.66745479140870e-05, ...
    2.04817376923090e-08,4.38706672844350e-07,-3.22776772385700e-05,-0.00150339245421480,-0.0406682535626490, ...
    -7.88473095593670e-10,1.27907178522850e-08,4.82253727185070e-07,2.29220763376610e-06,-1.67147664510610e-11, ...
    -0.00211714723213550,-23.8957419341040,-5.90595643242700e-18,-1.26218088991010e-06,-0.0389468424357390, ...
    1.12562113604590e-11,-8.23113408979980,1.98097128020880e-08,1.04069652101740e-19,-1.02347470959290e-13, ...
    -1.00181793795110e-09,-8.08829086469850e-11,0.106930318794090,-0.336622505741710,8.91858453554210e-25, ...
    3.06293168762320e-13,-4.20024676982080e-06,-5.90560296856390e-26,3.78269476134570e-06,-1.27686089346810e-15, ...
    7.30876105950610e-29,5.54147153507780e-17,-9.43697072412100e-07];
NRterms = 43;
IR = ones(dim,1)*IR;
JR = ones(dim,1)*JR;
nR = ones(dim,1)*nR;
pi = pi*ones(1,NRterms);
tau = tau*ones(1,NRterms);
dgammadpiR = sum(nR.*IR.*pi.^(IR-1).*(tau-0.5).^JR,2);
dgammadpi = dgammadpi0 + dgammadpiR;
end
function dgammadtautau = dgammadtautau2_pT(p,T)
dim = length(p);
pstar = 1; % [MPa] scaling pressure for nondimensional pressure, pi
Tstar = 540; % [K] scaling temperature for nondimensional temperature substitution variable
pi = p/pstar; % nondimensional pressure
tau = Tstar./T; % temperature substitution variable
%% ideal part
J0 = [0,1,-5,-4,-3,-2,-1,2,3]; % ideal part exponenets
n0 = [-9.69276865002170,10.0866559680180,-0.00560879112830200,0.0714527380814550,-0.407104982239280,1.42408191714440, ...
    -4.38395113194500,-0.284086324607720,0.0212684637533070];
N0terms = 9; % number of ideal terms in summation
J0 = ones(dim,1)*J0;
n0 = ones(dim,1)*n0;
tau0 = tau*ones(1,N0terms);
dgammadtautau0 = sum(n0.*J0.*(J0-1).*tau0.^(J0-2),2); % summation terms
%% residual part
IR = [1,1,1,1,1,2,2,2,2,2,3,3,3,3,3,4,4,4,5,6,6,6,7,7,7,8,8,9,10,10,10,16,16,18,20,20,20,21,22,23,24,24,24];
JR = [0,1,2,3,6,1,2,4,7,36,0,1,3,6,35,1,2,3,7,3,16,35,0,11,25,8,36,13,4,10,14,29,50,57,20,35,48,21,53,39,26,40,58];
nR = [-0.00177317424732130,-0.0178348622923580,-0.0459960136963650,-0.0575812590834320,-0.0503252787279300, ...
    -3.30326416702030e-05,-0.000189489875163150,-0.00393927772433550,-0.0437972956505730,-2.66745479140870e-05, ...
    2.04817376923090e-08,4.38706672844350e-07,-3.22776772385700e-05,-0.00150339245421480,-0.0406682535626490, ...
    -7.88473095593670e-10,1.27907178522850e-08,4.82253727185070e-07,2.29220763376610e-06,-1.67147664510610e-11, ...
    -0.00211714723213550,-23.8957419341040,-5.90595643242700e-18,-1.26218088991010e-06,-0.0389468424357390, ...
    1.12562113604590e-11,-8.23113408979980,1.98097128020880e-08,1.04069652101740e-19,-1.02347470959290e-13, ...
    -1.00181793795110e-09,-8.08829086469850e-11,0.106930318794090,-0.336622505741710,8.91858453554210e-25, ...
    3.06293168762320e-13,-4.20024676982080e-06,-5.90560296856390e-26,3.78269476134570e-06,-1.27686089346810e-15, ...
    7.30876105950610e-29,5.54147153507780e-17,-9.43697072412100e-07];
NRterms = 43;
IR = ones(dim,1)*IR;
JR = ones(dim,1)*JR;
nR = ones(dim,1)*nR;
pi = pi*ones(1,NRterms);
tauR = tau*ones(1,NRterms);
dgammadtautauR = sum(nR.*pi.^IR.*JR.*(JR-1).*(tauR-0.5).^(JR-2),2);
dgammadtautau = dgammadtautau0 + dgammadtautauR;
end
function dgammadpitau = dgammadpitau2_pT(p,T)
dim = length(p);
pstar = 1; % [MPa] scaling pressure for nondimensional pressure, pi
Tstar = 540; % [K] scaling temperature for nondimensional temperature substitution variable
pi = p/pstar; % nondimensional pressure
tau = Tstar./T; % temperature substitution variable
%% ideal part
dgammadpitau0 = 0;
%% residual part
IR = [1,1,1,1,1,2,2,2,2,2,3,3,3,3,3,4,4,4,5,6,6,6,7,7,7,8,8,9,10,10,10,16,16,18,20,20,20,21,22,23,24,24,24];
JR = [0,1,2,3,6,1,2,4,7,36,0,1,3,6,35,1,2,3,7,3,16,35,0,11,25,8,36,13,4,10,14,29,50,57,20,35,48,21,53,39,26,40,58];
nR = [-0.00177317424732130,-0.0178348622923580,-0.0459960136963650,-0.0575812590834320,-0.0503252787279300, ...
    -3.30326416702030e-05,-0.000189489875163150,-0.00393927772433550,-0.0437972956505730,-2.66745479140870e-05, ...
    2.04817376923090e-08,4.38706672844350e-07,-3.22776772385700e-05,-0.00150339245421480,-0.0406682535626490, ...
    -7.88473095593670e-10,1.27907178522850e-08,4.82253727185070e-07,2.29220763376610e-06,-1.67147664510610e-11, ...
    -0.00211714723213550,-23.8957419341040,-5.90595643242700e-18,-1.26218088991010e-06,-0.0389468424357390, ...
    1.12562113604590e-11,-8.23113408979980,1.98097128020880e-08,1.04069652101740e-19,-1.02347470959290e-13, ...
    -1.00181793795110e-09,-8.08829086469850e-11,0.106930318794090,-0.336622505741710,8.91858453554210e-25, ...
    3.06293168762320e-13,-4.20024676982080e-06,-5.90560296856390e-26,3.78269476134570e-06,-1.27686089346810e-15, ...
    7.30876105950610e-29,5.54147153507780e-17,-9.43697072412100e-07];
NRterms = 43;
IR = ones(dim,1)*IR;
JR = ones(dim,1)*JR;
nR = ones(dim,1)*nR;
pi = pi*ones(1,NRterms);
tau = tau*ones(1,NRterms);
dgammadpitauR = sum(nR.*IR.*pi.^(IR-1).*JR.*(tau-0.5).^(JR-1),2);
dgammadpitau = dgammadpitau0 + dgammadpitauR;
end
function dphidtau = dphidtau3_rhoT(rho,T)
dim = length(T);
Tc = 647.096; % [K] critical point temperature
rhoc = 322; % [kg/m^3] critical point density
tau = Tc./T;
delta = rho/rhoc;
I = [0,0,0,0,0,0,0,1,1,1,1,2,2,2,2,2,2,3,3,3,3,3,4,4,4,4,5,5,5,6,6,6,7,8,9,9,10,10,11];
J = [0,1,2,7,10,12,23,2,6,15,17,0,2,6,7,22,26,0,2,4,16,26,0,2,4,26,1,3,26,0,2,26,2,26,2,26,0,1,26];
n = [-15.7328452902390,20.9443969743070,-7.68677078787160,2.61859477879540,-2.80807811486200,1.20533696965170, ...
    -0.00845668128125020,-1.26543154777140,-1.15244078066810,0.885210439843180,-0.642077651816070,0.384934601866710, ...
    -0.852147088242060,4.89722815418770,-3.05026172569650,0.0394205368791540,0.125584084243080,-0.279993296987100, ...
    1.38997995694600,-2.01899150235700,-0.00821476371739630,-0.475960357349230,0.0439840744735000,-0.444764354287390, ...
    0.905720707197330,0.705224500879670,0.107705126263320,-0.329136232589540,-0.508710620411580,-0.0221754008730960, ...
    0.0942607516650920,0.164362784479610,-0.0135033722413480,-0.0148343453524720,0.000579229536280840, ...
    0.00323089047037110,8.09648029962150e-05,-0.000165576797950370,-4.49238990618150e-05];
Nterms = 39;
I = ones(dim,1)*I;
J = ones(dim,1)*J;
n = ones(dim,1)*n;
delta = delta*ones(1,Nterms);
tau = tau*ones(1,Nterms);
dphidtau = sum(n.*delta.^I.*J.*tau.^(J-1),2);
end
function dphiddelta = dphiddelta3_rhoT(rho,T)
dim = length(T);
Tc = 647.096; % [K] critical point temperature
rhoc = 322; % [kg/m^3] critical point density
tau = Tc./T;
delta = rho/rhoc;
I = [0,0,0,0,0,0,0,1,1,1,1,2,2,2,2,2,2,3,3,3,3,3,4,4,4,4,5,5,5,6,6,6,7,8,9,9,10,10,11];
J = [0,1,2,7,10,12,23,2,6,15,17,0,2,6,7,22,26,0,2,4,16,26,0,2,4,26,1,3,26,0,2,26,2,26,2,26,0,1,26];
n = [-15.7328452902390,20.9443969743070,-7.68677078787160,2.61859477879540,-2.80807811486200,1.20533696965170, ...
    -0.00845668128125020,-1.26543154777140,-1.15244078066810,0.885210439843180,-0.642077651816070,0.384934601866710, ...
    -0.852147088242060,4.89722815418770,-3.05026172569650,0.0394205368791540,0.125584084243080,-0.279993296987100, ...
    1.38997995694600,-2.01899150235700,-0.00821476371739630,-0.475960357349230,0.0439840744735000,-0.444764354287390, ...
    0.905720707197330,0.705224500879670,0.107705126263320,-0.329136232589540,-0.508710620411580,-0.0221754008730960, ...
    0.0942607516650920,0.164362784479610,-0.0135033722413480,-0.0148343453524720,0.000579229536280840, ...
    0.00323089047037110,8.09648029962150e-05,-0.000165576797950370,-4.49238990618150e-05];
Nterms = 39;
n0 = 1.065807002851300; % prexponential constant
I = ones(dim,1)*I;
J = ones(dim,1)*J;
n = ones(dim,1)*n;
deltaND = delta*ones(1,Nterms);
tau = tau*ones(1,Nterms);
dphiddelta = n0./delta + sum(n.*I.*deltaND.^(I-1).*tau.^J,2);
end
function dphidtautau = dphidtautau3_rhoT(rho,T)
dim = length(T);
Tc = 647.096; % [K] critical point temperature
rhoc = 322; % [kg/m^3] critical point density
tau = Tc./T;
delta = rho/rhoc;
I = [0,0,0,0,0,0,0,1,1,1,1,2,2,2,2,2,2,3,3,3,3,3,4,4,4,4,5,5,5,6,6,6,7,8,9,9,10,10,11];
J = [0,1,2,7,10,12,23,2,6,15,17,0,2,6,7,22,26,0,2,4,16,26,0,2,4,26,1,3,26,0,2,26,2,26,2,26,0,1,26];
n = [-15.7328452902390,20.9443969743070,-7.68677078787160,2.61859477879540,-2.80807811486200,1.20533696965170, ...
    -0.00845668128125020,-1.26543154777140,-1.15244078066810,0.885210439843180,-0.642077651816070,0.384934601866710, ...
    -0.852147088242060,4.89722815418770,-3.05026172569650,0.0394205368791540,0.125584084243080,-0.279993296987100, ...
    1.38997995694600,-2.01899150235700,-0.00821476371739630,-0.475960357349230,0.0439840744735000,-0.444764354287390, ...
    0.905720707197330,0.705224500879670,0.107705126263320,-0.329136232589540,-0.508710620411580,-0.0221754008730960, ...
    0.0942607516650920,0.164362784479610,-0.0135033722413480,-0.0148343453524720,0.000579229536280840, ...
    0.00323089047037110,8.09648029962150e-05,-0.000165576797950370,-4.49238990618150e-05];
Nterms = 39;
I = ones(dim,1)*I;
J = ones(dim,1)*J;
n = ones(dim,1)*n;
delta = delta*ones(1,Nterms);
tau = tau*ones(1,Nterms);
dphidtautau = sum(n.*delta.^I.*J.*(J-1).*tau.^(J-2),2);
end
function dphiddeltatau = dphiddeltatau3_rhoT(rho,T)
dim = length(T);
Tc = 647.096; % [K] critical point temperature
rhoc = 322; % [kg/m^3] critical point density
tau = Tc./T;
delta = rho/rhoc;
I = [0,0,0,0,0,0,0,1,1,1,1,2,2,2,2,2,2,3,3,3,3,3,4,4,4,4,5,5,5,6,6,6,7,8,9,9,10,10,11];
J = [0,1,2,7,10,12,23,2,6,15,17,0,2,6,7,22,26,0,2,4,16,26,0,2,4,26,1,3,26,0,2,26,2,26,2,26,0,1,26];
n = [-15.7328452902390,20.9443969743070,-7.68677078787160,2.61859477879540,-2.80807811486200,1.20533696965170, ...
    -0.00845668128125020,-1.26543154777140,-1.15244078066810,0.885210439843180,-0.642077651816070,0.384934601866710, ...
    -0.852147088242060,4.89722815418770,-3.05026172569650,0.0394205368791540,0.125584084243080,-0.279993296987100, ...
    1.38997995694600,-2.01899150235700,-0.00821476371739630,-0.475960357349230,0.0439840744735000,-0.444764354287390, ...
    0.905720707197330,0.705224500879670,0.107705126263320,-0.329136232589540,-0.508710620411580,-0.0221754008730960, ...
    0.0942607516650920,0.164362784479610,-0.0135033722413480,-0.0148343453524720,0.000579229536280840, ...
    0.00323089047037110,8.09648029962150e-05,-0.000165576797950370,-4.49238990618150e-05];
Nterms = 39;
I = ones(dim,1)*I;
J = ones(dim,1)*J;
n = ones(dim,1)*n;
delta = delta*ones(1,Nterms);
tau = tau*ones(1,Nterms);
dphiddeltatau = sum(n.*I.*delta.^(I-1).*J.*tau.^(J-1),2);
end
function dphiddeltadelta = dphiddeltadelta3_rhoT(rho,T)
dim = length(T);
Tc = 647.096; % [K] critical point temperature
rhoc = 322; % [kg/m^3] critical point density
tau = Tc./T;
delta = rho/rhoc;
I = [0,0,0,0,0,0,0,1,1,1,1,2,2,2,2,2,2,3,3,3,3,3,4,4,4,4,5,5,5,6,6,6,7,8,9,9,10,10,11];
J = [0,1,2,7,10,12,23,2,6,15,17,0,2,6,7,22,26,0,2,4,16,26,0,2,4,26,1,3,26,0,2,26,2,26,2,26,0,1,26];
n = [-15.7328452902390,20.9443969743070,-7.68677078787160,2.61859477879540,-2.80807811486200,1.20533696965170, ...
    -0.00845668128125020,-1.26543154777140,-1.15244078066810,0.885210439843180,-0.642077651816070,0.384934601866710, ...
    -0.852147088242060,4.89722815418770,-3.05026172569650,0.0394205368791540,0.125584084243080,-0.279993296987100, ...
    1.38997995694600,-2.01899150235700,-0.00821476371739630,-0.475960357349230,0.0439840744735000,-0.444764354287390, ...
    0.905720707197330,0.705224500879670,0.107705126263320,-0.329136232589540,-0.508710620411580,-0.0221754008730960, ...
    0.0942607516650920,0.164362784479610,-0.0135033722413480,-0.0148343453524720,0.000579229536280840, ...
    0.00323089047037110,8.09648029962150e-05,-0.000165576797950370,-4.49238990618150e-05];
Nterms = 39;
n0 = 1.065807002851300; % prexponential constant
I = ones(dim,1)*I;
J = ones(dim,1)*J;
n = ones(dim,1)*n;
deltaND = delta*ones(1,Nterms);
tau = tau*ones(1,Nterms);
dphiddeltadelta = -n0./delta.^2 + sum(n.*I.*(I-1).*deltaND.^(I-2).*tau.^J,2);
end
function dTsatdpsat = dTsatdpsat_p(p)
pstar = 1; % [Mpa]
Tstar = 1; % [K]
n = [1167.05214527670;-724213.167032060;-17.0738469400920;12020.8247024700;-3232555.03223330;14.9151086135300; ...
    -4823.26573615910;405113.405420570;-0.238555575678490;650.175348447980];
beta = (p/pstar).^0.25;
E = beta.^2 + n(3)*beta + n(6);
F = n(1)*beta.^2 + n(4)*beta + n(7);
G = n(2)*beta.^2 + n(5)*beta + n(8);
D = 2*G./(-F - (F.^2 - 4*E.*G).^0.5);
dbetadp = 1./(4*pstar*beta.^3);
n11 = 4*E.*G;
discriminant = (F.^2 - n11).^0.5;
n12 = F+discriminant;
n13 = n12.^2;
dDdE = -4*G.^2./(discriminant.*n13);
dEdbeta = 2*beta + n(3);
dDdF = 2*G.*(F./discriminant + 1)./n13;
dFdbeta = 2*n(1)*beta + n(4);
dDdG = -2./n12 - n11./(discriminant.*n13);
dGdbeta = 2*n(2)*beta + n(5);
n14 = D - n(10);
ddthetadD = (1 - n14./((n14.^2 - 4*n(9)).^0.5))/2;
dTsatdpsat = Tstar*ddthetadD.*(dDdE.*dEdbeta + dDdF.*dFdbeta + dDdG.*dGdbeta).*dbetadp;
end
%% backward and boundary functions
function T = T1_ph(p,h) % [K]
dim = length(p);
pstar = 1; % [MPa]
Tstar = 1; % [K]
hstar = 2500; % [kJ/kg]
pi = p/pstar;
eta = h/hstar;
I = [0,0,0,0,0,0,1,1,1,1,1,1,1,2,2,3,3,4,5,6];
J = [0,1,2,6,22,32,0,1,2,3,4,10,32,10,32,10,32,32,32,32];
n = [-238.724899245210,404.211886379450,113.497468817180,-5.84576160480390,-0.000152854824131400,-1.08667076953770e-06, ...
    -13.3917448726020,43.2110391835590,-54.0100671705060,30.5358922039160,-6.59647494236380,0.00939654008783630, ...
    1.15736475053400e-07,-2.58586412820730e-05,-4.06443630847990e-09,6.64561861916350e-08,8.06707341030270e-11, ...
    -9.34777712139470e-13,5.82654420206010e-15,-1.50201859535030e-17];
Nterms = 20;
I = ones(dim,1)*I;
J = ones(dim,1)*J;
n = ones(dim,1)*n;
pi = pi*ones(1,Nterms);
eta = eta*ones(1,Nterms);
theta = sum(n.*pi.^I.*(eta+1).^J,2);
T = Tstar*theta;
end
function T = T2a_ph(p,h) % [K]
dim = length(p);
pstar = 1; % [MPa]
Tstar = 1; % [K]
hstar = 2000; % [kJ/kg]
pi = p/pstar;
eta = h/hstar;
Ia = [0,0,0,0,0,0,1,1,1,1,1,1,1,1,1,2,2,2,2,2,2,2,2,3,3,4,4,4,5,5,5,6,6,7];
Ja = [0,1,2,3,7,20,0,1,2,3,7,9,11,18,44,0,2,7,36,38,40,42,44,24,44,12,32,44,32,36,42,34,44,28];
na = [1089.89523182880,849.516544955350,-107.817480918260,33.1536548012630,-7.42320167902480,11.7650487243560, ...
    1.84457493557900,-4.17927005496240,6.24781969358120,-17.3445631081140,-200.581768620960,271.960654737960, ...
    -455.113182858180,3091.96886047550,252266.403578720,-0.00617074228683390,-0.310780466295830,11.6708730771070, ...
    128127984.040460,-985549096.232760,2822454697.30020,-3594897141.07030,1722734991.31970,-13551.3342407750, ...
    12848734.6646500,1.38657242832260,235988.325565140,-13105236.5450540,7399.98354747660,-551966.970300600, ...
    3715408.59962330,19127.7292396600,-415351.648356340,-62.4598551925070];
Naterms = 34;
Ia = ones(dim,1)*Ia;
Ja = ones(dim,1)*Ja;
na = ones(dim,1)*na;
pi = pi*ones(1,Naterms);
eta = eta*ones(1,Naterms);
theta = sum(na.*pi.^Ia.*(eta-2.1).^Ja,2);
T = Tstar*theta;
end
function T = T2b_ph(p,h) % [K]
dim = length(p);
pstar = 1; % [MPa]
Tstar = 1; % [K]
hstar = 2000; % [kJ/kg]
pi = p/pstar;
eta = h/hstar;
Ib = [0,0,0,0,0,0,0,0,1,1,1,1,1,1,1,1,2,2,2,2,3,3,3,3,4,4,4,4,4,4,5,5,5,6,7,7,9,9];
Jb = [0,1,2,12,18,24,28,40,0,2,6,12,18,24,28,40,2,8,18,40,1,2,12,24,2,12,18,24,28,40,18,24,40,28,2,28,1,40];
nb = [1489.50410795160,743.077983140340,-97.7083187978370,2.47424647056740,-0.632813200160260,1.13859521296580, ...
    -0.478118636486250,0.00852081234315440,0.937471473779320,3.35931186049160,3.38093556014540,0.168445396719040, ...
    0.738757452366950,-0.471287374361860,0.150202731397070,-0.00217641142197500,-0.0218107553247610,-0.108297844036770, ...
    -0.0463333246358120,7.12803519595510e-05,0.000110328317899990,0.000189552483879020,0.00308915411605370, ...
    0.00135555045549490,2.86402374774560e-07,-1.07798573575120e-05,-7.64627124548140e-05,1.40523928183160e-05, ...
    -3.10838143314340e-05,-1.03027382121030e-06,2.82172816350400e-07,1.27049022719450e-06,7.38033534682920e-08, ...
    -1.10301392389090e-08,-8.14563652078330e-14,-2.51805456829620e-11,-1.75652339694070e-18,8.69341563441630e-15];
Nbterms = 38;
Ib = ones(dim,1)*Ib;
Jb = ones(dim,1)*Jb;
nb = ones(dim,1)*nb;
pi = pi*ones(1,Nbterms);
eta = eta*ones(1,Nbterms);
theta = sum(nb.*(pi-2).^Ib.*(eta-2.6).^Jb,2);
T = Tstar*theta;
end
function T = T2c_ph(p,h) % [K]
dim = length(p);
pstar = 1; % [MPa]
Tstar = 1; % [K]
hstar = 2000; % [kJ/kg]
pi = p/pstar;
eta = h/hstar;
Ic = [-7,-7,-6,-6,-5,-5,-2,-2,-1,-1,0,0,1,1,2,6,6,6,6,6,6,6,6];
Jc = [0,4,0,2,0,2,0,1,0,2,0,1,4,8,4,0,1,4,10,12,16,20,22];
nc = [-3236839855524.20,7326335090218.10,358250899454.470,-583401318515.900,-10783068217.4700,20825544563.1710, ...
    610747.835645160,859777.225355800,-25745.7236041700,31081.0884227140,1208.23158659360,482.197551092550, ...
    3.79660012724860,-10.8429848800770,-0.0453641726766600,1.45591156586980e-13,1.12615974072300e-12,-1.78049822406860e-11, ...
    1.23245796908320e-07,-1.16069211309840e-06,2.78463670885540e-05,-0.000592700384741760,0.00129185829918780];
Ncterms = 23;
Ic = ones(dim,1)*Ic;
Jc = ones(dim,1)*Jc;
nc = ones(dim,1)*nc;
pi = pi*ones(1,Ncterms);
eta = eta*ones(1,Ncterms);
theta = sum(nc.*(pi+25).^Ic.*(eta-1.8).^Jc,2);
T = Tstar*theta;
end
function T = T3a_ph(p,h) % [K]
dim = length(p);
pstar = 100; % [MPa]
Tstar = 760; % [K]
hstar = 2300; % [kJ/kg]
pi = p/pstar;
eta = h/hstar;
I = [-12,-12,-12,-12,-12,-12,-12,-12,-10,-10,-10,-8,-8,-8,-8,-5,-3,-2,-2,-2,-1,-1,0,0,1,3,3,4,4,10,12];
J = [0,1,2,6,14,16,20,22,1,5,12,0,2,4,10,2,0,1,3,4,0,2,0,1,1,0,1,0,3,4,5];
n = [-1.33645667811215e-07,4.55912656802978e-06,-1.46294640700979e-05,0.00639341312970080,372.783927268847, ...
    -7186.54377460447,573494.752103400,-2675693.29111439,-3.34066283302614e-05,-0.0245479214069597,47.8087847764996, ...
    7.64664131818904e-06,0.00128350627676972,0.0171219081377331,-8.51007304583213,-0.0136513461629781, ...
    -3.84460997596657e-06,0.00337423807911655,-0.551624873066791,0.729202277107470,-0.00992522757376041, ...
    -0.119308831407288,0.793929190615421,0.454270731799386,0.209998591259910,-0.00642109823904738,-0.0235155868604540, ...
    0.00252233108341612,-0.00764885133368119,0.0136176427574291,-0.0133027883575669];
Nterms = 31;
I = ones(dim,1)*I;
J = ones(dim,1)*J;
n = ones(dim,1)*n;
pi = pi*ones(1,Nterms);
eta = eta*ones(1,Nterms);
theta = sum(n.*(pi+0.240).^I.*(eta-0.615).^J,2);
T = Tstar*theta;
end
function T = T3b_ph(p,h) % [K]
dim = length(p);
pstar = 100; % [MPa]
Tstar = 860; % [K]
hstar = 2800; % [kJ/kg]
pi = p/pstar;
eta = h/hstar;
I = [-12,-12,-10,-10,-10,-10,-10,-8,-8,-8,-8,-8,-6,-6,-6,-4,-4,-3,-2,-2,-1,-1,-1,-1,-1,-1,0,0,1,3,5,6,8];
J = [0,1,0,1,5,10,12,0,1,2,4,10,0,1,2,0,1,5,0,4,2,4,6,10,14,16,0,2,1,1,1,1,1];
n = [3.23254573644920e-05,-0.000127575556587181,-0.000475851877356068,0.00156183014181602,0.105724860113781, ...
    -85.8514221132534,724.140095480911,0.00296475810273257,-0.00592721983365988,-0.0126305422818666,-0.115716196364853, ...
    84.9000969739595,-0.0108602260086615,0.0154304475328851,0.0750455441524466,0.0252520973612982,-0.0602507901232996, ...
    -3.07622221350501,-0.0574011959864879,5.03471360939849,-0.925081888584834,3.91733882917546,-77.3146007130190, ...
    9493.08762098587,-1410437.19679409,8491662.30819026,0.861095729446704,0.323346442811720,0.873281936020439, ...
    -0.436653048526683,0.286596714529479,-0.131778331276228,0.00676682064330275];
Nterms = 33;
I = ones(dim,1)*I;
J = ones(dim,1)*J;
n = ones(dim,1)*n;
pi = pi*ones(1,Nterms);
eta = eta*ones(1,Nterms);
theta = sum(n.*(pi+0.298).^I.*(eta-0.720).^J,2);
T = Tstar*theta;
end
function v = v3a_ph(p,h) % [m^3/kg]
dim = length(p);
vstar = 0.0028; % [m^3/kg]
pstar = 100; % [MPa]
hstar = 2100; % [kJ/kg]
pi = p/pstar;
eta = h/hstar;
I = [-12,-12,-12,-12,-10,-10,-10,-8,-8,-6,-6,-6,-4,-4,-3,-2,-2,-1,-1,-1,-1,0,0,1,1,1,2,2,3,4,5,8];
J = [6,8,12,18,4,7,10,5,12,3,4,22,2,3,7,3,16,0,1,2,3,0,1,0,1,2,0,2,0,2,2,2];
n = [0.00529944062966028,-0.170099690234461,11.1323814312927,-2178.98123145125,-0.000506061827980875,0.556495239685324, ...
    -9.43672726094016,-0.297856807561527,93.9353943717186,0.0192944939465981,0.421740664704763,-3689141.26282330, ...
    -0.00737566847600639,-0.354753242424366,-1.99768169338727,1.15456297059049,5683.66875815960,0.00808169540124668, ...
    0.172416341519307,1.04270175292927,-0.297691372792847,0.560394465163593,0.275234661176914,-0.148347894866012, ...
    -0.0651142513478515,-2.92468715386302,0.0664876096952665,3.52335014263844,-0.0146340792313332,-2.24503486668184, ...
    1.10533464706142,-0.0408757344495612];
Nterms = 32;
I = ones(dim,1)*I;
J = ones(dim,1)*J;
n = ones(dim,1)*n;
pi = pi*ones(1,Nterms);
eta = eta*ones(1,Nterms);
omega = sum(n.*(pi+0.128).^I.*(eta-0.727).^J,2);
v = vstar*omega;
end
function v = v3b_ph(p,h) % [m^3/kg]
dim = length(p);
vstar = 0.0088; % [m^3/kg]
pstar = 100; % [MPa]
hstar = 2800; % [kJ/kg]
pi = p/pstar;
eta = h/hstar;
I = [-12,-12,-8,-8,-8,-8,-8,-8,-6,-6,-6,-6,-6,-6,-4,-4,-4,-3,-3,-2,-2,-1,-1,-1,-1,0,1,1,2,2];
J = [0,1,0,1,3,6,7,8,0,1,2,5,6,10,3,6,10,0,2,1,2,0,1,4,5,0,0,1,2,6];
n = [-2.25196934336318e-09,1.40674363313486e-08,2.33784085280560e-06,-3.31833715229001e-05,0.00107956778514318, ...
    -0.271382067378863,1.07202262490333,-0.853821329075382,-2.15214194340526e-05,0.000769656088222730, ...
    -0.00431136580433864,0.453342167309331,-0.507749535873652,-100.475154528389,-0.219201924648793,-3.21087965668917, ...
    607.567815637771,0.000557686450685932,0.187499040029550,0.00905368030448107,0.285417173048685,0.0329924030996098, ...
    0.239897419685483,4.82754995951394,-11.8035753702231,0.169490044091791,-0.0179967222507787,0.0371810116332674, ...
    -0.0536288335065096,1.60697101092520];
Nterms = 30;
I = ones(dim,1)*I;
J = ones(dim,1)*J;
n = ones(dim,1)*n;
pi = pi*ones(1,Nterms);
eta = eta*ones(1,Nterms);
omega = sum(n.*(pi+0.0661).^I.*(eta-0.720).^J,2);
v = vstar*omega;
end
function h = h2bc_p(p)
pstar = 1; % [MPa]
hstar = 1; % [kJ/kg]
pi = p/pstar;
n = [0.90584278514723e3;-0.67955786399241;0.12809002730136e-3;0.26526571908428e4;0.45257578905948e1];
eta = n(4) + ((pi-n(5))/n(3)).^0.5;
h = eta*hstar;
end
function h = h3ab_p(p)
pstar = 1; % [MPa]
hstar = 1; % [kJ/kg]
pi = p/pstar;
n = [0.201464004206875e4;0.374696550136983e1;-0.219921901054187e-1;0.875131686009950e-4];
eta = n(1) + pi.*(n(2) + pi.*(n(3) + pi*n(4))); % use Horner's Method to speed up calculations
h = eta*hstar;
end
function T = TB23_p(p)
pstar = 1; % [MPa]
Tstar = 1; % [K]
pi = p/pstar;
n = [0.34805185628969e3; -0.11671859879975e1; 0.10192970039326e-2; 0.57254459862746e3; 0.13918839778870e2];
theta = n(4) + ((pi-n(5))/n(3)).^0.5;
T = theta*Tstar;
end
function p = p3sat_h(h)
dim = length(h);
pstar = 22; % [MPa]
hstar = 2600; % [kJ/kg]
eta = h/hstar;
I = [0,1,1,1,1,5,7,8,14,20,22,24,28,36];
J = [0,1,3,4,36,3,0,24,16,16,3,18,8,24];
n = [0.600073641753024,-9.36203654849857,24.6590798594147,-107.014222858224,-91582131580576.8,-8623.32011700662, ...
    -23.5837344740032,2.52304969384128e+17,-3.89718771997719e+18,-3.33775713645296e+22,35649946963.6328, ...
    -1.48547544720641e+26,3.30611514838798e+18,8.13641294467829e+37];
Nterms = 14;
I = ones(dim,1)*I;
J = ones(dim,1)*J;
n = ones(dim,1)*n;
eta = eta*ones(1,Nterms);
pi = sum(n.*(eta-1.02).^I.*(eta-0.608).^J,2);
p = pstar*pi;
end
function v = v3c_pT(p,T)
dim = length(p);
Table4 = [0.00220000000000000,40,690,35,0.259000000000000,0.903000000000000,1,1,1];
vstar = Table4(1);pstar = Table4(2);Tstar = Table4(3); Nterms = Table4(4);
a = Table4(5);b = Table4(6);c = Table4(7);d = Table4(8);e = Table4(9);
pi = p/pstar;theta = T/Tstar;
TableA1_3 = [-12,6,3.11967788763030;-12,8,27671.3458847564;-12,10,32258310.3403269;-10,6,-342.416065095363; ...
    -10,8,-899732.529907377;-10,10,-79389204.9821251;-8,5,95.3193003217388;-8,6,2297.84742345072;-8,7,175336.675322499; ...
    -6,8,7912143.65222792;-5,1,3.19933345844209e-05;-5,4,-65.9508863555767;-5,7,-833426.563212851; ...
    -4,2,0.0645734680583292;-4,8,-3820310.20570813;-3,0,4.06398848470079e-05;-3,3,31.0327498492008; ...
    -2,0,-0.000892996718483724;-2,4,234.604891591616;-2,5,3775.15668966951;-1,0,0.0158646812591361; ...
    -1,1,0.707906336241843;-1,2,12.6016225146570;0,0,0.736143655772152;0,1,0.676544268999101;0,2,-17.8100588189137; ...
    1,0,-0.156531975531713;1,2,11.7707430048158;2,0,0.0840143653860447;2,1,-0.186442467471949;2,3,-44.0170203949645; ...
    2,7,1232904.23502494;3,0,-0.0240650039730845;3,7,-1070777.16660869;8,1,0.0438319858566475];
I = ones(dim,1)*TableA1_3(:,1)'; J = ones(dim,1)*TableA1_3(:,2)'; n = ones(dim,1)*TableA1_3(:,3)';
pi = pi*ones(1,Nterms);
theta = theta*ones(1,Nterms);
omega = (sum(n.*((pi-a).^c).^I.*((theta-b).^d).^J,2)).^e;
v = vstar*omega;
end
function v = v3r_pT(p,T)
dim = length(p);
Table4 = [0.00540000000000000,23,650,27,0.874000000000000,0.982000000000000,1,1,1];
vstar = Table4(1);pstar = Table4(2);Tstar = Table4(3); Nterms = Table4(4);
a = Table4(5);b = Table4(6);c = Table4(7);d = Table4(8);e = Table4(9);
pi = p/pstar;theta = T/Tstar;
TableA1_18 = [-8,6,0.00144165955660863;-8,14,-7014385996282.58;-3,-3,-8.30946716459219e-17;-3,3,0.261975135368109; ...
    -3,4,393.097214706245;-3,5,-10433.4030654021;-3,8,490112654.154211;0,-1,-0.000147104222772069; ...
    0,0,1.03602748043408;0,1,3.05308890065089;0,5,-3997452.76971264;3,-6,5.69233719593750e-12; ...
    3,-2,-0.0464923504407778;8,-12,-5.35400396512906e-18;8,-10,3.99988795693162e-13;8,-8,-5.36479560201811e-07; ...
    8,-5,0.0159536722411202;10,-12,2.70303248860217e-15;10,-10,2.44247453858506e-08;10,-8,-9.83430636716454e-06; ...
    10,-6,0.0663513144224454;10,-5,-9.93456957845006;10,-4,546.491323528491;10,-3,-14336.5406393758; ...
    10,-2,150764.974125511;12,-12,-3.37209709340105e-10;14,-12,3.77501980025469e-09];
I = ones(dim,1)*TableA1_18(:,1)'; J = ones(dim,1)*TableA1_18(:,2)'; n = ones(dim,1)*TableA1_18(:,3)';
pi = pi*ones(1,Nterms);
theta = theta*ones(1,Nterms);
omega = (sum(n.*((pi-a).^c).^I.*((theta-b).^d).^J,2)).^e;
v = vstar*omega;
end
function v = v3s_pT(p,T)
dim = length(p);
Table4 = [0.00220000000000000,21,640,29,0.886000000000000,0.990000000000000,1,1,4];
vstar = Table4(1);pstar = Table4(2);Tstar = Table4(3); Nterms = Table4(4);
a = Table4(5);b = Table4(6);c = Table4(7);d = Table4(8);e = Table4(9);
pi = p/pstar;theta = T/Tstar;
TableA1_19 = [-12,20,-5.32466612140254e+22;-12,24,1.00415480000824e+31;-10,22,-1.91540001821367e+29; ...
    -8,14,1.05618377808847e+16;-6,36,2.02281884477061e+58;-5,8,88458547.2596134;-5,16,1.66540181638363e+22; ...
    -4,6,-313563.197669111;-4,32,-1.85662327545324e+53;-3,3,-0.0624942093918942;-3,8,-5041607241.32590; ...
    -2,4,18751.4491833092;-1,1,0.00121399979993217;-1,2,1.88317043049455;-1,3,-1670.73503962060; ...
    0,0,0.965961650599775;0,1,2.94885696802488;0,4,-65391.5627346115;0,28,6.04012200163444e+49; ...
    1,0,-0.198339358557937;1,32,-1.75984090163501e+57;3,0,3.56314881403987;3,1,-575.991255144384; ...
    3,2,45621.3415338071;4,3,-10917404.4987829;4,18,4.37796099975134e+33;4,24,-6.16552611135792e+45; ...
    5,4,1935687689.17797;14,24,9.50898170425042e+53];
I = ones(dim,1)*TableA1_19(:,1)'; J = ones(dim,1)*TableA1_19(:,2)'; n = ones(dim,1)*TableA1_19(:,3)';
pi = pi*ones(1,Nterms);
theta = theta*ones(1,Nterms);
omega = (sum(n.*((pi-a).^c).^I.*((theta-b).^d).^J,2)).^e;
v = vstar*omega;
end
function v = v3t_pT(p,T)
dim = length(p);
Table4 = [0.00880000000000000,20,650,33,0.803000000000000,1.02000000000000,1,1,1];
vstar = Table4(1);pstar = Table4(2);Tstar = Table4(3); Nterms = Table4(4);
a = Table4(5);b = Table4(6);c = Table4(7);d = Table4(8);e = Table4(9);
pi = p/pstar;theta = T/Tstar;
TableA1_20 = [0,0,1.55287249586268;0,1,6.64235115009031;0,4,-2893.66236727210;0,12,-3859232023098.48; ...
    1,0,-2.91002915783761;1,10,-829088246858.083;2,0,1.76814899675218;2,6,-534686695.713469; ...
    2,14,1.60464608687834e+17;3,3,196435.366560186;3,8,1566374275417.29;4,0,-1.78154560260006; ...
    4,10,-2.29746237623692e+15;7,3,38565900.1648006;7,4,1105544467.90543;7,7,-67707383068734.9; ...
    7,20,-3.27910592086523e+30;7,36,-3.41552040860644e+50;10,10,-5.27251339709047e+20;10,12,2.45375640937055e+23; ...
    10,14,-1.68776617209269e+26;10,16,3.58958955867578e+28;10,22,-6.56475280339411e+35;18,18,3.55286045512301e+38; ...
    20,32,5.69021454413270e+57;22,22,-7.00584546433113e+47;22,36,-7.05772623326374e+64;24,24,1.66861176200148e+52; ...
    28,28,-3.00475129680486e+60;32,22,-6.68481295196808e+50;32,32,4.28432338620678e+68;32,36,-4.44227367758304e+71; ...
    36,36,-2.81396013562745e+76];
I = ones(dim,1)*TableA1_20(:,1)'; J = ones(dim,1)*TableA1_20(:,2)'; n = ones(dim,1)*TableA1_20(:,3)';
pi = pi*ones(1,Nterms);
theta = theta*ones(1,Nterms);
omega = (sum(n.*((pi-a).^c).^I.*((theta-b).^d).^J,2)).^e;
v = vstar*omega;
end
function v = v3u_pT(p,T)
dim = length(p);
Table12 = [0.00260000000000000,23,650,38,0.902000000000000,0.988000000000000,1,1,1];
vstar = Table12(1);pstar = Table12(2);Tstar = Table12(3); Nterms = Table12(4);
a = Table12(5);b = Table12(6);c = Table12(7);d = Table12(8);e = Table12(9);
pi = p/pstar;theta = T/Tstar;
TableA2_1 = [-12,14,1.22088349258355e+17;-10,10,1042164686.08488;-10,12,-8.82666931564652e+15; ...
    -10,14,2.59929510849499e+19;-8,10,222612779142211;-8,12,-8.78473585050085e+17;-8,14,-3.14432577551552e+21; ...
    -6,8,-2169349169962.85;-6,12,1.59079648196849e+20;-5,4,-339.567617303423;-5,8,8843876513378.36; ...
    -5,12,-8.43405926846418e+20;-3,2,11.4178193518022;-1,-1,-0.000122708229235641;-1,1,-106.201671767107; ...
    -1,12,9.03443213959313e+24;-1,14,-6.93996270370852e+27;0,-3,6.48916718965575e-09;0,1,7189.57567127851; ...
    1,-2,0.00105581745346187;2,5,-651903203602581;2,10,-1.60116813274676e+24;3,-5,-5.10254294237837e-09; ...
    5,-4,-0.152355388953402;5,2,677143292290.144;5,3,276378438378930;6,-5,0.0116862983141686;6,2,-30142694798017.1; ...
    8,-8,1.69719813884840e-08;8,8,1.04674840020929e+26;10,-4,-10801.6904560140;12,-12,-9.90623601934295e-13; ...
    12,-4,5361164.83602738;12,4,2.26145963747881e+21;14,-12,-4.88731565776210e-10;14,-10,1.51001548880670e-05; ...
    14,-6,-22770.0464643920;14,6,-7.81754507698846e+27];
I = ones(dim,1)*TableA2_1(:,1)'; J = ones(dim,1)*TableA2_1(:,2)'; n = ones(dim,1)*TableA2_1(:,3)';
pi = pi*ones(1,Nterms);
theta = theta*ones(1,Nterms);
omega = (sum(n.*((pi-a).^c).^I.*((theta-b).^d).^J,2)).^e;
v = vstar*omega;
end
function v = v3x_pT(p,T)
dim = length(p);
Table12 = [0.00490000000000000,23,650,36,0.910000000000000,0.988000000000000,1,1,1];
vstar = Table12(1);pstar = Table12(2);Tstar = Table12(3); Nterms = Table12(4);
a = Table12(5);b = Table12(6);c = Table12(7);d = Table12(8);e = Table12(9);
pi = p/pstar;theta = T/Tstar;
TableA2_4 = [-8,14,3.77373741298151e+18;-6,10,-5071008837229.13;-5,10,-1.03363225598860e+15; ...
    -4,1,1.84790814320773e-06;-4,2,-0.000924729378390945;-4,14,-4.25999562292738e+23;-3,-2,-4.62307771873973e-13; ...
    -3,12,1.07319065855767e+21;-1,5,64866249228.0682;0,0,2.44200600688281;0,4,-8515357334.84258; ...
    0,10,1.69894481433592e+21;1,-10,2.15780222509020e-27;1,-1,-0.320850551367334;2,6,-3.82642448458610e+16; ...
    3,-12,-2.75386077674421e-29;3,0,-563199.253391666;3,8,-3.26068646279314e+20;4,3,39794900155318.4; ...
    5,-6,1.00824008584757e-07;5,-2,16223.4569738433;5,1,-43235522531.9745;6,1,-592874245598.610; ...
    8,-6,1.33061647281106;8,-3,1573381.97797544;8,1,25818961427085.3;8,8,2.62413209706358e+24; ...
    10,-8,-0.0920011937431142;12,-10,0.00220213765905426;12,-8,-11.0433759109547;12,-5,8470048.70612087; ...
    12,-4,-592910695.762536;14,-12,-1.83027173269660e-05;14,-10,0.181339603516302;14,-8,-1192.28759669889; ...
    14,-6,4308676.58061468];
I = ones(dim,1)*TableA2_4(:,1)'; J = ones(dim,1)*TableA2_4(:,2)'; n = ones(dim,1)*TableA2_4(:,3)';
pi = pi*ones(1,Nterms);
theta = theta*ones(1,Nterms);
omega = (sum(n.*((pi-a).^c).^I.*((theta-b).^d).^J,2)).^e;
v = vstar*omega;
end
function v = v3y_pT(p,T)
dim = length(p);
Table12 = [0.00310000000000000,22,650,20,0.996000000000000,0.994000000000000,1,1,4];
vstar = Table12(1);pstar = Table12(2);Tstar = Table12(3); Nterms = Table12(4);
a = Table12(5);b = Table12(6);c = Table12(7);d = Table12(8);e = Table12(9);
pi = p/pstar;theta = T/Tstar;
TableA2_5 = [0,-3,-5.25597995024633e-10;0,1,5834.41305228407;0,5,-1.34778968457925e+16;0,8,1.18973500934212e+25; ...
    1,8,-1.59096490904708e+26;2,-4,-3.15839902302021e-07;2,-1,496.212197158239;2,4,3.27777227273171e+18; ...
    2,5,-5.27114657850696e+21;3,-8,2.10017506281863e-17;3,4,7.05106224399834e+20;3,8,-2.66713136106469e+30; ...
    4,-6,-1.45370512554562e-08;4,6,1.49333917053130e+27;5,-2,-14979562.0287641;5,1,-3.81881906271100e+15; ...
    8,-8,7.24660165585797e-05;8,-2,-93780816955019.3;10,-5,5144114683.76383;12,-8,-82819.8594040141];
I = ones(dim,1)*TableA2_5(:,1)'; J = ones(dim,1)*TableA2_5(:,2)'; n = ones(dim,1)*TableA2_5(:,3)';
pi = pi*ones(1,Nterms);
theta = theta*ones(1,Nterms);
omega = (sum(n.*((pi-a).^c).^I.*((theta-b).^d).^J,2)).^e;
v = vstar*omega;
end
function v = v3z_pT(p,T)
dim = length(p);
Table12 = [0.00380000000000000,22,650,23,0.993000000000000,0.994000000000000,1,1,4];
vstar = Table12(1);pstar = Table12(2);Tstar = Table12(3); Nterms = Table12(4);
a = Table12(5);b = Table12(6);c = Table12(7);d = Table12(8);e = Table12(9);
pi = p/pstar;theta = T/Tstar;
TableA2_6 = [-8,3,2.44007892290650e-11;-6,6,-4630574.30331242;-5,6,7288032747.77712;-5,8,3.27776302858856e+15; ...
    -4,5,-1105981701.18409;-4,6,-3238999157299.57;-4,8,9.23814007023245e+15;-3,-2,8.42250080413712e-13; ...
    -3,5,663221436245.506;-3,6,-167170186672139;-2,2,2537.49358701391;-1,-6,-8.19731559610523e-21; ...
    0,3,328380587890.663;1,1,-62500479.1171543;2,6,8.03197957462023e+20;3,-6,-2.04397011338353e-11; ...
    3,-2,-3783.91047055938;6,-6,0.00972876545938620;6,-5,15.4355721681459;6,-4,-3739.62862928643; ...
    6,-1,-68285901137.4572;8,-8,-0.000248488015614543;8,-4,3945360.49497068];
I = ones(dim,1)*TableA2_6(:,1)'; J = ones(dim,1)*TableA2_6(:,2)'; n = ones(dim,1)*TableA2_6(:,3)';
pi = pi*ones(1,Nterms);
theta = theta*ones(1,Nterms);
omega = (sum(n.*((pi-a).^c).^I.*((theta-b).^d).^J,2)).^e;
v = vstar*omega;
end


function df = diffx(f, x0,y0 )
    % 输入参数说明：
    % f: 目标函数句柄
    % x0: 求导点坐标（向量形式，如[p,h]）
    % h0: 初始步长（默认1e-3）
    % tol: 收敛容差（默认1e-6）
    h0=1e-3;
    tol=1e-6;
    max_iter=100;
    D = zeros(max_iter,1); % 存储各次迭代结果
    h = h0;
    for k = 1:max_iter
        % 中心差分计算
        df_forward = (f(x0 + h/2,y0) - f(x0 - h/2,y0)) / h;
        df_half = (f(x0 + h/4,y0) - f(x0 - h/4,y0)) / (h/2);
        
        % Richardson外推
        D(k) = (4*df_half - df_forward)/3;
        
        % 误差控制
        if k>1 && abs(D(k)-D(k-1)) < tol
            break;
        end
        h = h/2; % 自动缩小步长
    end
    df = D(k);
    if df ==0
        df=( f(x0+h0 ,y0)-f(x0,y0))/h0;
    end
end


function df = diffy(f, x0,y0 )
    % 输入参数说明：
    % f: 目标函数句柄
    % x0: 求导点坐标（向量形式，如[p,h]）
    % h0: 初始步长（默认1e-3）
    % tol: 收敛容差（默认1e-6）
    h0=1e-3;
    tol=1e-6;
    max_iter=100;
    D = zeros(max_iter,1); % 存储各次迭代结果
    h = h0;
    for k = 1:max_iter
        % 中心差分计算
        df_forward = (f(x0,y0 + h/2) - f(x0,y0 - h/2)) / h;
        df_half = (f(x0,y0 + h/4) - f(x0,y0 - h/4)) / (h/2);
        
        % Richardson外推
        D(k) = (4*df_half - df_forward)/3;
        
        % 误差控制
        if k>1 && abs(D(k)-D(k-1)) < tol
            break;
        end
        h = h/2; % 自动缩小步长
    end
    df = D(k);
    if df ==0
        df=( f(x0 ,y0+h0)-f(x0,y0))/h0;
    end
end

function df = diff1(f, x0 )
    % 输入参数说明：
    % f: 目标函数句柄
    % x0: 求导点坐标（向量形式，如[p,h]）
    % h0: 初始步长（默认1e-3）
    % tol: 收敛容差（默认1e-6）
    h0=1e-3;
    tol=1e-6;
    max_iter=100;
    D = zeros(max_iter,1); % 存储各次迭代结果
    h = h0;
    for k = 1:max_iter
        % 中心差分计算
        df_forward = (f(x0 + h/2) - f(x0 - h/2)) / h;
        df_half = (f(x0 + h/4) - f(x0 - h/4)) / (h/2);
        
        % Richardson外推
        D(k) = (4*df_half - df_forward)/3;
        
        % 误差控制
        if k>1 && abs(D(k)-D(k-1)) < tol
            break;
        end
        h = h/2; % 自动缩小步长
    end
    df = D(k);
end
